simulink model "Quazi_square"  (R2023a)
settings: Solver=ode23tb  StartTime=0.0  StopTime=1  MaxStep=1e-4  RelTol=1e-3
libraries: spsMosfetLib x4, simulink x2, spsDCVoltageSourceLib x1, spsSeriesRLCBranchLib x1, spsVoltageMeasurementLib x1, spspowerguiLib x1
settings Model: Creator=gaming3  LastModifiedBy=gaming3

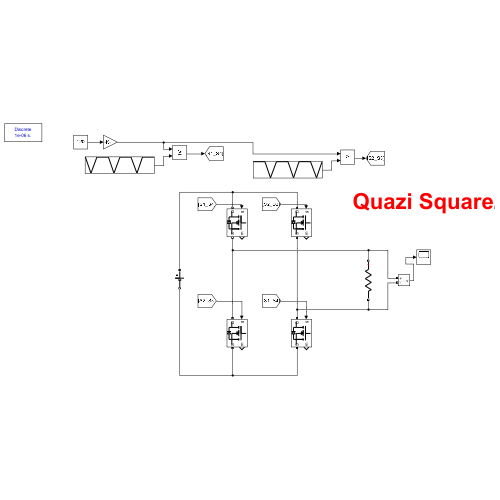
[thumbnail: Simulink's stored preview of the top-level diagram]
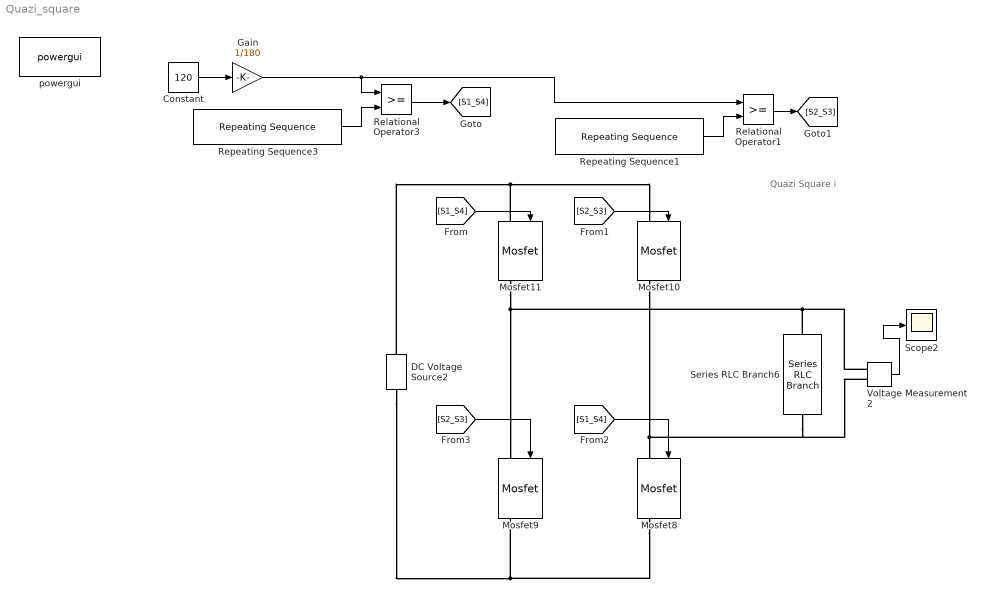
== system Quazi_square ==
  note: Quazi Square i
  Constant : Constant  Value=120
  DC Voltage Source2 : spsDCVoltageSourceLib/DC Voltage Source  Amplitude=310  Measurements=None
  Gain : Gain  Gain=1/180
  Mosfet{8..11} (4 alike) : spsMosfetLib/Mosfet  Ron=0.1  Lon=0  Rd=0.01  Vfd=0  IC=0  Rs=1e5  Cs=inf  Measurements=on
  Relational Operator1 : RelationalOperator  OutDataTypeStr=boolean  RndMeth=Simplest  InputSameDT=off
  Relational Operator3 : RelationalOperator  OutDataTypeStr=boolean  RndMeth=Simplest  InputSameDT=off
  Repeating Sequence1 : simulink/Sources/Repeating Sequence  rep_seq_t=[0 0.01 0.01001 (3*0.02)/4 0.02 ]  rep_seq_y=[1.001 1.001 1 0 1]
  Repeating Sequence3 : simulink/Sources/Repeating Sequence  rep_seq_t=[0 0.02/4 0.02/2 0.01001 0.02]  rep_seq_y="[1 0 1  1.001  1.001]"
  Scope2 : Scope
  Series RLC Branch6 : spsSeriesRLCBranchLib/Series RLC Branch  LConnTagsString=__new0  RConnTagsString=__new0  BranchType=R  Resistance=100  Inductance=1e-3  SetiL0=off  InitialCurrent=0  Capacitance=1e-6  Setx0=off  InitialVoltage=0  Measurements=None
  Voltage Measurement2 : spsVoltageMeasurementLib/Voltage Measurement  PhasorSimulation=off  OutputType=Complex  PSBequivalent=0
  powergui : spspowerguiLib/powergui  Priority=1  SimulationMode=Discrete  SampleTime=1e-06  frequency=60  Iterations=50  frequencyindice=0  Pbase=100e6  ErrMax=1e-4  UnitsV=kV  UnitsW=MW  buscounter=0  FunctionMessages=off  echomessages=off  EnableUseOfTLC=off  CurrentSourceSwitches=off  DisableSnubberDevices=off  DisableRonSwitches=off  DisableVfSwitches=off  DisplayEquations=off  AutomaticDiscreteSolvers=off  SolverType=Tustin/Backward Euler (TBE)  Interpol=off  ExternalGateDelay=off  methode=off  Ts=100  x0status=blocks  SPID=on  SwTol=0  HookPort=off  NonlinearTolerance=1e-4  nMaxIteration=100  ContinueOnMaxIteration=off  RestoreLinks=warning  ResistiveCurrentMeasurement=off  Frange=[0:2:500]  Ylog=off  Xlog=on  ShowGrid=off  save=off  variable=ZData  structure=0  ZoomFFT=off  StartTime=0.0  cycles=1  DisplayStyle=1  fundamental=60  FreqAxis=off  MaxFrequency=1000  frequencyindicesteady=1  RmsSteady=1  display=off
  wires:
  Voltage Measurement2/1 -> Scope2/1
  Repeating Sequence3/1 -> Relational Operator3/2
  Gain/1 -> Relational Operator1/1, Relational Operator3/1
  Constant/1 -> Gain/1
  Repeating Sequence1/1 -> Relational Operator1/2
  Relational Operator1/1 -> [S2_S3]
  Relational Operator3/1 -> [S1_S4]
  [S1_S4] -> Mosfet8/1
  [S1_S4] -> Mosfet11/1
  [S2_S3] -> Mosfet10/1
  [S2_S3] -> Mosfet9/1
  connections:
  Series RLC Branch6/LConn1 -- Mosfet9/LConn1 -- Mosfet11/RConn1 -- Voltage Measurement2/LConn1
  Mosfet10/RConn1 -- Mosfet8/LConn1 -- Voltage Measurement2/LConn2 -- Series RLC Branch6/RConn1
  DC Voltage Source2/RConn1 -- Mosfet11/LConn1 -- Mosfet10/LConn1
  Mosfet8/RConn1 -- Mosfet9/RConn1 -- DC Voltage Source2/LConn1
